simulink model "HSD_model"  (R2019b)
settings: Solver=FixedStepAuto  StartTime=0  StopTime=500  RelTol=1e-3  EnableMultiTasking=on
undefined symbols (not defined in the file or in its folder): gray
libraries: visiontextngfix x2
settings Model: EnablePacing=on  Creator=DreamChaser  LastModifiedBy=ARES
settings SolverCC: AutoInsertRateTranBlk=on
settings DataIOCC: SaveOutput=off  SaveTime=off  ReturnWorkspaceOutputs=off
settings DebuggingCC: ArithmeticOperatorsInVariantConditions=warning
settings SFSimCC: SimUseLocalCustomCode=off  CustomCodeUndefinedFunction=UseInterfaceOnly
settings RTWCC: RTWUseLocalCustomCode=off
settings CodeAppCC: StateflowObjectComments=on

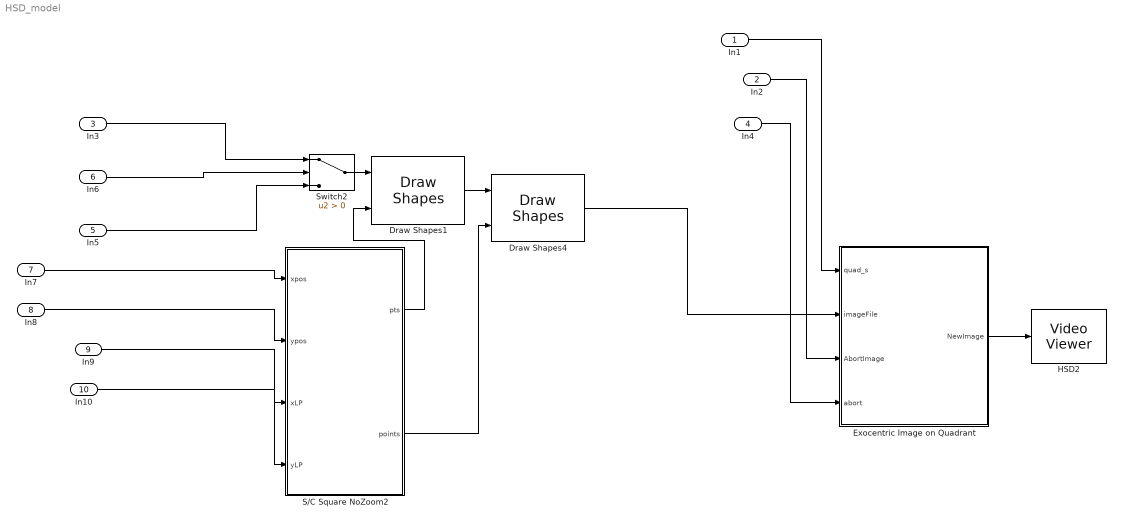
== system HSD_model ==
  In1 : Inport  OutDataTypeStr=double  PortDimensions=1
  In2 : Inport  Port=2  OutDataTypeStr=int32  PortDimensions=[524 700 3]
  In3 : Inport  Port=3  OutDataTypeStr=int32  PortDimensions=[1124 1124 3]
  In4 : Inport  Port=4  OutDataTypeStr=double  PortDimensions=1
  In5 : Inport  Port=5  OutDataTypeStr=int32  PortDimensions=[1124 1124 3]
  In6 : Inport  Port=6  OutDataTypeStr=boolean  PortDimensions=1
  In7 : Inport  Port=7  OutDataTypeStr=double  PortDimensions=1
  In8 : Inport  Port=8  OutDataTypeStr=double  PortDimensions=1  SampleTime=1
  In9 : Inport  Port=9  OutDataTypeStr=double  PortDimensions=1
  In10 : Inport  Port=10  OutDataTypeStr=double  PortDimensions=1
  Draw Shapes1 : visiontextngfix/Draw Shapes  shape=Rectangles  fill=off  lineWidth=3  fillClrSource=Specify via dialog  display=User-specified value  intensity=200  color=[2147483648 1073741824 2147483648]  opacity=1  viewport=Entire image  antialiasing=off  inType=Obsolete  imagePorts=One multidimensional signal  roundingMode=Floor  overflowMode=off  memoryMode=Specify word length  memoryWordLength=16  prodOutputMode=Binary point scaling  prodOutputWordLength=32  prodOutputFracLength=14  prodOutputSlope=2^-14  accumSlope=2^-14  memoryFracLength=14
      settings: SourceProductName=Computer Vision Toolbox
  Draw Shapes4 : visiontextngfix/Draw Shapes  shape=Polygons  fill=off  lineWidth=2  fillClrSource=Specify via dialog  display=User-specified value  intensity=200  color=[2147483648 2147483648 0]  opacity=1.0  viewport=Entire image  antialiasing=off  inType=Obsolete  imagePorts=One multidimensional signal  roundingMode=Floor  overflowMode=off  memoryMode=Specify word length  memoryWordLength=16  prodOutputMode=Binary point scaling  prodOutputWordLength=32  prodOutputFracLength=14  prodOutputSlope=2^-14  accumSlope=2^-14  memoryFracLength=14
      settings: SourceProductName=Computer Vision Toolbox
  Exocentric Image on Quadrant : MATLAB Function  TreatAsAtomicUnit=on
  HSD2 : VideoViewer  colormapValue=gray(256)  FigPos=[-2047 1278 1024 1230]
  S/C Square NoZoom2 : MATLAB Function  TreatAsAtomicUnit=on
  Switch2 : Switch  Criteria=u2 > Threshold
  wires:
  In8/1 -> S/C Square NoZoom2/2(ypos)
  S/C Square NoZoom2/1(pts) -> Draw Shapes1/2
  In10/1 -> S/C Square NoZoom2/4(yLP)
  In4/1 -> Exocentric Image on Quadrant/4(abort)
  Switch2/1 -> Draw Shapes1/1
  Draw Shapes1/1 -> Draw Shapes4/1
  S/C Square NoZoom2/2(points) -> Draw Shapes4/2
  Exocentric Image on Quadrant/1(NewImage) -> HSD2/1
  In3/1 -> Switch2/1
  In6/1 -> Switch2/2
  Draw Shapes4/1 -> Exocentric Image on Quadrant/2(imageFile)
  In1/1 -> Exocentric Image on Quadrant/1(quad_s)
  In9/1 -> S/C Square NoZoom2/3(xLP)
  In7/1 -> S/C Square NoZoom2/1(xpos)
  In2/1 -> Exocentric Image on Quadrant/3(AbortImage)
  In5/1 -> Switch2/3

== matlab function HSD_model/S//C Square NoZoom2 ==
  settings: sampleTime=1.0
  data: xpos input; pts output; points output; ypos input; xLP input; yLP input
%%%%%%%%%%%%%%%%%%%%%%%%%%%%%%%%%%%%%
% This function is used to define the pixel points of the landing site
% and s/c position. 
% WHEN YOU DEFINE THE ACTUAL SHAPES THE NUMBER OF POINTS MUST BE THE SAME!!
% Elliott Davis 
% Edited: 4/30/18
% 
% Nicholas Miller
% Adjusting to accomodate circles for both the S/C and the LP position.
% Edited: 6/21/19
%%%%%%%%%%%%%%%%%%%%%%%%%%%%%%%%%%%%%

function [pts,points] = fcn( xpos,ypos,xLP,yLP)

%% Define size of shapes
numPixels = 1124;
feetPixels = 24000/numPixels;
%terrain = 0; %What does this do? -nick

%% Define color of shapes
% color 255,255,0 = 
% color 255,0,255 = 

color = int32([25,0,0; 0,0,50]);

%% Convert from feet to pixels
xPixel = xpos/feetPixels;
yPixel = numPixels-(ypos/feetPixels);
xPixel_LP = xLP/feetPixels;
yPixel_LP = numPixels-(yLP/feetPixels);
squareSize = 12;  % Pixels, Originally 6
radius = 15; % Pixels, Originally 7

%% Define s/c position points
p2 = [ xPixel+(squareSize/2) yPixel+(squareSize/2)...
       xPixel-(squareSize/2) yPixel+(squareSize/2)... 
       xPixel-(squareSize/2) yPixel-(squareSize/2)...
       xPixel+(squareSize/2) yPixel-(squareSize/2)...
       xPixel+(squareSize/2) yPixel+(squareSize/2) ];
%p2 = [xPixel yPixel squareSize-1];
    
    
%% Define landing site points
% p3 = [ xPixel_LP-(squareSize/2)+x_shift yPixel_LP+(squareSize/2)+y_shift...
%        xPixel_LP+(squareSize/2)+x_shift yPixel_LP+(squareSize/2)+y_shift...
%        xPixel_LP+(squareSize/2)+x_shift yPixel_LP-(squareSize/2)+y_shift...
%        xPixel_LP+x_shift                yPixel_LP-squareSize+y_shift...
%        xPixel_LP-(squareSize/2)+x_shift yPixel_LP-(squareSize/2)+y_shift];

% p3 = [(xPixel_LP - (radius/2)) (yPixel_LP -(radius/2)) xPixel_LP yPixel_LP...
%      ; (xPixel_LP + (radius/2)) (yPixel_LP +(radius/2)) xPixel_LP yPIxel_LP]; %
%p3 = [xPixel_LP yPixel_LP radius]; %Landing Point Circle
 p3 = [(xPixel_LP - (radius/2)) (yPixel_LP -(radius/2)) radius radius]; %
% Landing point square

%% Output points
pts = int32(p3);
points = int32(p2);

== matlab function HSD_model/Exocentric Image on Quadrant ==
  settings: sampleTime=1.0
  data: quad_s input; imageFile input; NewImage output size=[1628 1628 3]; AbortImage input; abort input
%%%%%%%%%%%%%%%%%%%%%%%%%%%%%%%%%%%%%
% This function moves the terrain map with the movement of the s/c
% position. Assure that the feet per pixel and number of pixels is the same
% as Define ALD Pts function.
% Elliott Davis 
% Edited: 4/30/18
% Adapted to only show quadrant from an exocentric perspective
% Abort Image and failure detection image
% Edited: 7/25/19 by Nicholas Miller
%%%%%%%%%%%%%%%%%%%%%%%%%%%%%%%%%%%%%

function NewImage = fcn(quad_s, imageFile, AbortImage, abort)

% Define the number of pixels in the terrain mapnumPixels = 350;

% Define the feet per each pixel
numPixels = 1124;
feetPixels = 24000/numPixels;
pixelTotal = 1124; %Specific value for image size Ex: 713x713 pixels

if quad_s == 1
    xPixel = int32(pixelTotal*0.75);
    yPixel = int32(pixelTotal*0.25);
elseif quad_s == 2
    xPixel = int32(pixelTotal*0.25);
    yPixel = int32(pixelTotal*0.25);
elseif quad_s == 3
    xPixel = int32(pixelTotal*0.25);
    yPixel = int32(pixelTotal*(0.75));
else
    xPixel = int32(pixelTotal*0.75);
    yPixel = int32(pixelTotal*(0.75));
end
    
% Convert from feet to pixels for the s/c position
% xPixel = int32(xpos/feetPixels);
% yPixel =int32(numPixels-(ypos/feetPixels));

% Define the size of the map that you want to see.
%viewingSize = 178.25; %Pixels
 viewingSize = 500; %Pixels
%% Define the maximum and minimum points on the map
xLow = xPixel-viewingSize*1.25; %makes it rectangular
xHigh = xPixel+viewingSize*1.25;
% xLow = xPixel-viewingSize/2; %makes it square
% xHigh = xPixel+viewingSize/2;
yLow = yPixel-viewingSize;
yHigh = yPixel+viewingSize;

%% Assure that if you are getting close to edges the map stops moving
if xLow < 1
    xLow = int32(1);
end 

if xHigh > pixelTotal
    xHigh = int32(pixelTotal);
end

if yLow < 1
    yLow = int32(1);
end 

if yHigh > pixelTotal
    yHigh = int32(pixelTotal);
end

%% Attempting to change image prior to sim end (PLEASE DO NOT ERASE)
% if StopSim(1)==1
%     NewImage = AbortImage;
%     
% elseif StopSim(2)==1
%     Roll_angle = abs(roll);  % Max +/-6 deg/s
%     Pitch_angle = abs(pitch);  % Max +/-6 deg/s
% %     V_north =VN.data(end);
% %     V_east = VE.data(end);
%     V_mag = sqrt(Vn^2 + Ve^2); % Max 4 ft/s
% %     Des_Vel=hdot.data(end);
%     
%     if V_mag>4 || Roll_angle>6 ||Pitch_angle>6 || Desc<-8
%          NewImage = CrashImage;
%     else
%         NewImage = SuccessImage;
%     end
%     
% elseif StopSim(3)==1 && h~=0
%     NewImage = CrashImage;
% else
%     % Output the defined image size
%     NewImage = imageFile(yLow:yHigh,xLow:xHigh,1:3);
% end

% if abort==1
%     NewImage=AbortImage;
% else
     NewImage = imageFile;%(yLow:yHigh,xLow:xHigh,1:3);
% end

% if fail_button == 1
%     NewImage = ButtonPressImage; % Display the "Failure Detected" image
% end

NewImage=int32(NewImage);
